simulink model "BMO_codegen"  (R2015b)
settings: Solver=FixedStepAuto  StartTime=0.0  StopTime=inf  FixedStep=BMOk_stepSize  RelTol=1e-3  SampleTimeConstraint=STIndependent
undefined symbols (not defined in the file): BMOk_BatteryCurrentThresh, BMOk_CcClosing, BMOk_CcOpening, BMOk_Charging, BMOk_ChargingSleep, BMOk_Discharging, BMOk_Off, BMOk_On, BMOk_PowerClosed, BMOk_PowerOff, BMOk_PowerOn
libraries: simulink x2
settings Model: Creator=nctzv8  LastModifiedBy=nctzv8
settings ConfigSet: Description=OpenECU configuration set for code generation under RTW-EC.
settings SolverCC: PositivePriorityOrder=on
settings DataIOCC: SaveFormat=Array  SignalLoggingSaveFormat=ModelDataLogs
settings OptimizationCC: DefaultParameterBehavior=Inlined  InlineInvariantSignals=on  ExpressionDepthLimit=2147483647  StateBitsets=on  DataBitsets=on  ZeroExternalMemoryAtStartup=off  ZeroInternalMemoryAtStartup=off  NoFixptDivByZeroProtection=on  EfficientFloat2IntCast=on  OptimizeModelRefInitCode=on  LifeSpan=1
settings DebuggingCC: SaveWithParameterizedLinksMsg=none  UnderspecifiedInitializationDetection=Classic  MergeDetectMultiDrivingBlocksExec=none  SignalResolutionControl=TryResolveAllWithWarning  MultiTaskDSMMsg=warning  MultiTaskCondExecSysMsg=none  SingleTaskRateTransMsg=error  CheckMatrixSingularityMsg=warning  VectorMatrixConversionMsg=warning  FcnCallInpInsideContextMsg=UseLocalSettings  SignalLabelMismatchMsg=warning  StateNameClashWarn=warning
settings HardwareCC: ProdBitPerPointer=32  ProdLargestAtomicInteger=Long  ProdLargestAtomicFloat=Double  ProdEndianess=BigEndian  ProdWordSize=32  ProdHWDeviceType=Freescale->32-bit PowerPC  TargetIntDivRoundTo=Zero  TargetEndianess=BigEndian  TargetHWDeviceType=Freescale->32-bit PowerPC  ProdEqTarget=off
settings RTWCC: SystemTargetFile=openecu_ert.tlc  MakeCommand=make_rtw optimized_floating_point=1  TemplateMakefile=openecu_ert_r2015b_64.tmf  Description=OpenECU Platform Target (ERT, optimised floating-point code)  RetainRTWFile=on  IncludeHyperlinkInReport=on
settings CodeAppCC: ForceParamTrailComments=on  IgnoreCustomStorageClasses=off  SimulinkDataObjDesc=on  CustomSymbolStrType=$N$R$M  InsertBlockDesc=on  InternalIdentifier=Classic
settings STFCustomTargetCC: TargetLibSuffix=.a  GenerateSampleERTMain=on  ConcurrentExecutionCompliant=off  IncludeMdlTerminateFcn=off  GeneratePreprocessorConditionals=Use local settings  CombineOutputUpdateFcns=on  IncludeFileDelimiter=UseQuote  ERTCustomFileBanners=on  SupportContinuousTime=off  MATLABClassNameForMDSCustomization=Simulink.SoftwareTarget.ERTCustomization  CPPClassGenCompliant=off  GRTInterface=off  SystemTargetFile=openecu_ert.tlc
settings ERTTargetCC: GenerateSampleERTMain=on  ParMdlRefBuildCompliant=off  CompOptLevelCompliant=off  ConcurrentExecutionCompliant=off  IncludeMdlTerminateFcn=off  ERTFirstTimeCompliant=off  IncludeFileDelimiter=UseQuote  SupportNonInlinedSFcns=on  ModelStepFunctionPrototypeControlCompliant=off  CPPClassGenCompliant=off  UseToolchainInfoCompliant=off  ExtModeMexFile=noextcomm  InlinedParameterPlacement=NonHierarchical  ERTSrcFileBannerTemplate=oe_code_c_template.cgt  ERTHdrFileBannerTemplate=oe_code_h_template.cgt  ERTDataSrcFileTemplate=oe_data_c_template.cgt  ERTDataHdrFileTemplate=oe_data_h_template.cgt  ERTCustomFileTemplate=example_file_process.tlc  GlobalDataDefinition=InSeparateSourceFile  GlobalDataReference=InSeparateHeaderFile  EnableUserReplacementTypes=on

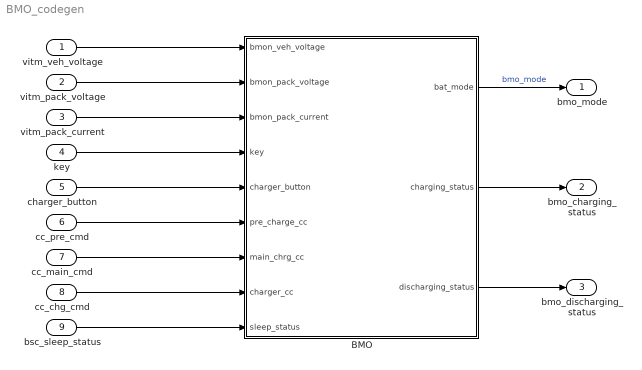
== system BMO_codegen ==
  vitm_veh_voltage : Inport
  vitm_pack_voltage : Inport  Port=2
  vitm_pack_current : Inport  Port=3
  key : Inport  Port=4  OutDataTypeStr=uint8
  charger_button : Inport  Port=5  OutDataTypeStr=uint8
  cc_pre_cmd : Inport  Port=6
  cc_main_cmd : Inport  Port=7
  cc_chg_cmd : Inport  Port=8  OutDataTypeStr=boolean
  bsc_sleep_status : Inport  Port=9  OutDataTypeStr=boolean
  BMO : Subsystem  TreatAsAtomicUnit=on
  bmo_mode : Outport
  bmo_charging_status : Outport  Port=2
  bmo_discharging_status : Outport  Port=3
  wires:
  vitm_veh_voltage/1 -> BMO/1(bmon_veh_voltage)
  vitm_pack_voltage/1 -> BMO/2(bmon_pack_voltage)
  vitm_pack_current/1 -> BMO/3(bmon_pack_current)
  key/1 -> BMO/4(key)
  cc_pre_cmd/1 -> BMO/6(pre_charge_cc)
  BMO/1(bat_mode) -> bmo_mode/1  "bmo_mode"
  BMO/2(charging_status) -> bmo_charging_status/1
  BMO/3(discharging_status) -> bmo_discharging_status/1
  bsc_sleep_status/1 -> BMO/9(sleep_status)
  cc_chg_cmd/1 -> BMO/8(charger_cc)
  cc_main_cmd/1 -> BMO/7(main_chrg_cc)
  charger_button/1 -> BMO/5(charger_button)

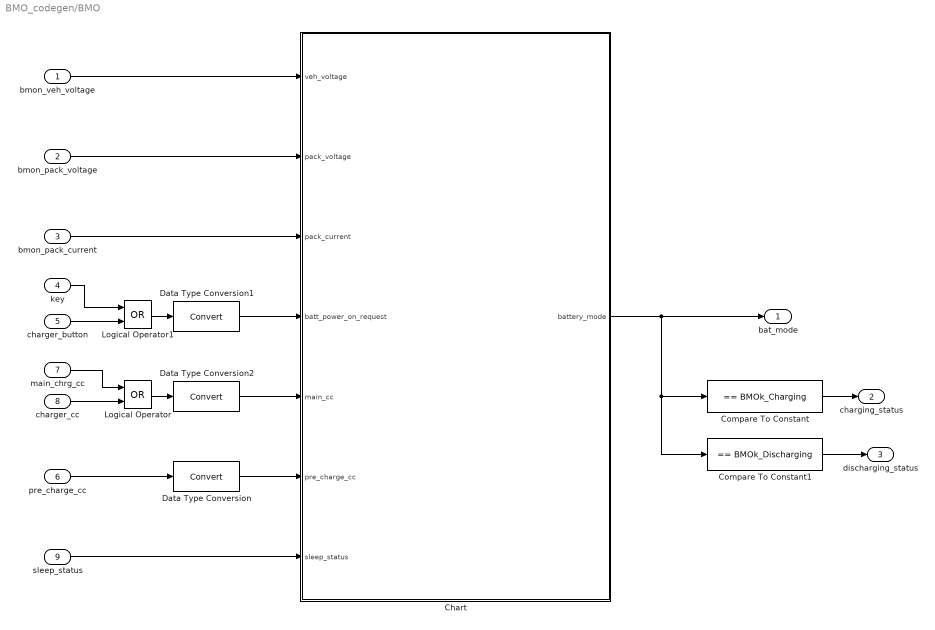
== system BMO_codegen/BMO ==
  bmon_veh_voltage : Inport
  bmon_pack_voltage : Inport  Port=2
  bmon_pack_current : Inport  Port=3
  key : Inport  Port=4
  charger_button : Inport  Port=5
  pre_charge_cc : Inport  Port=6
  main_chrg_cc : Inport  Port=7
  charger_cc : Inport  Port=8
  sleep_status : Inport  Port=9
  Chart : Stateflow chart  TreatAsAtomicUnit=on
  Compare To Constant : simulink/Logic and Bit Operations/Compare To Constant  relop===  const=BMOk_Charging  OutDataTypeStr=boolean
  Compare To Constant1 : simulink/Logic and Bit Operations/Compare To Constant  relop===  const=BMOk_Discharging  OutDataTypeStr=boolean
  Data Type Conversion : DataTypeConversion
  Data Type Conversion1 : DataTypeConversion
  Data Type Conversion2 : DataTypeConversion
  Logical Operator : Logic  Operator=OR  AllPortsSameDT=off  OutDataTypeStr=boolean
  Logical Operator1 : Logic  Operator=OR  AllPortsSameDT=off  OutDataTypeStr=boolean
  bat_mode : Outport
  charging_status : Outport  Port=2
  discharging_status : Outport  Port=3
  wires:
  pre_charge_cc/1 -> Data Type Conversion/1
  Compare To Constant/1 -> charging_status/1
  bmon_pack_voltage/1 -> Chart/2(pack_voltage)
  bmon_veh_voltage/1 -> Chart/1(veh_voltage)
  bmon_pack_current/1 -> Chart/3(pack_current)
  Data Type Conversion/1 -> Chart/6(pre_charge_cc)
  Data Type Conversion2/1 -> Chart/5(main_cc)
  Compare To Constant1/1 -> discharging_status/1
  Chart/1(battery_mode) -> Compare To Constant1/1, Compare To Constant/1, bat_mode/1
  sleep_status/1 -> Chart/7(sleep_status)
  Logical Operator/1 -> Data Type Conversion2/1
  main_chrg_cc/1 -> Logical Operator/1
  charger_cc/1 -> Logical Operator/2
  Logical Operator1/1 -> Data Type Conversion1/1
  charger_button/1 -> Logical Operator1/2
  key/1 -> Logical Operator1/1
  Data Type Conversion1/1 -> Chart/4(batt_power_on_request)

== stateflow chart BMO_codegen/BMO/Chart ==
  state Power_OFF
    entry:
    battery_mode = BMOk_PowerOff;
  state Charging_Sleep
    entry:
    battery_mode = BMOk_ChargingSleep;
  state Power_ON
    entry:
    battery_mode = BMOk_PowerOn;
  state Opening_Contactors
    entry:
    battery_mode = BMOk_CcOpening;
  state Closing_Contactors
    entry:
    battery_mode = BMOk_CcClosing;
  state Closing_MainContactors
    entry:
    battery_mode = BMOk_CcClosing;
  state Power_Closed
    state Power_Closed_Default
      entry:
      battery_mode = BMOk_PowerClosed;
    state Discharging
      entry:
      battery_mode = BMOk_Discharging;
    state Charging
      entry:
      battery_mode = BMOk_Charging;
    (default) -> Power_Closed_Default
    Power_Closed_Default -> (junction 28)
    (junction 28) -> Power_Closed_Default [order 3]
    (junction 28) -> Discharging [order 1] : [pack_current < -BMOk_BatteryCurrentThresh]
    (junction 28) -> Charging [order 2] : [pack_current > BMOk_BatteryCurrentThresh]
    Discharging -> (junction 28)
    Charging -> (junction 28)
  (default) -> Power_OFF
  Opening_Contactors -> Power_OFF [order 1] : [batt_power_on_request == BMOk_Off]
  Power_OFF -> Power_ON : [batt_power_on_request == BMOk_On]
  Power_ON -> Power_OFF [order 2] : [batt_power_on_request == BMOk_Off]
  Power_ON -> Charging_Sleep [order 4] : [sleep_status ==1]
  Opening_Contactors -> Power_ON [order 2] : [main_cc == BMOk_Off]
  Charging_Sleep -> Power_ON : [sleep_status ==0]
  Power_ON -> Closing_MainContactors [order 3] : [main_cc == BMOk_On]
  (junction 43) -> Opening_Contactors : [main_cc == BMOk_Off]
  Power_ON -> Closing_Contactors [order 1] : [pre_charge_cc == BMOk_On]
  Closing_Contactors -> Power_Closed : [main_cc == BMOk_On]
  Power_Closed -> (junction 43)
  Closing_MainContactors -> Power_Closed
  data: battery_mode output uint8; BMOk_PowerOff parameter uint8; BMOk_PowerOn parameter uint8; BMOk_CcClosing parameter uint8; BMOk_CcOpening parameter uint8; BMOk_PowerClosed parameter uint8; BMOk_Discharging parameter uint8; BMOk_Charging parameter uint8; veh_voltage input double; pack_voltage input double; pack_current input double; batt_power_on_request input uint8; BMOk_BatteryCurrentThresh parameter double; BMOk_On parameter uint8; BMOk_Off parameter uint8; main_cc input boolean; pre_charge_cc input boolean; sleep_status input boolean; BMOk_ChargingSleep parameter uint8
